simulink model "LowPassFilter_TEST"  (R2020a)
settings: Solver=VariableStepAuto  StartTime=0.0  StopTime=10.0  RelTol=1e-3
settings Model: Creator=109813  LastModifiedBy=109813

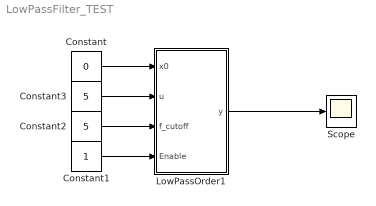
== system LowPassFilter_TEST ==
  Constant : Constant  Value=0
  Constant1 : Constant
  Constant2 : Constant  Value=5
  Constant3 : Constant  Value=5
  LowPassOrder1 : Subsystem
  Scope : Scope
  wires:
  Constant/1 -> LowPassOrder1/1(x0)
  Constant1/1 -> LowPassOrder1/4(Enable)
  Constant2/1 -> LowPassOrder1/3(f_cutoff)
  Constant3/1 -> LowPassOrder1/2(u)
  LowPassOrder1/1(y) -> Scope/1

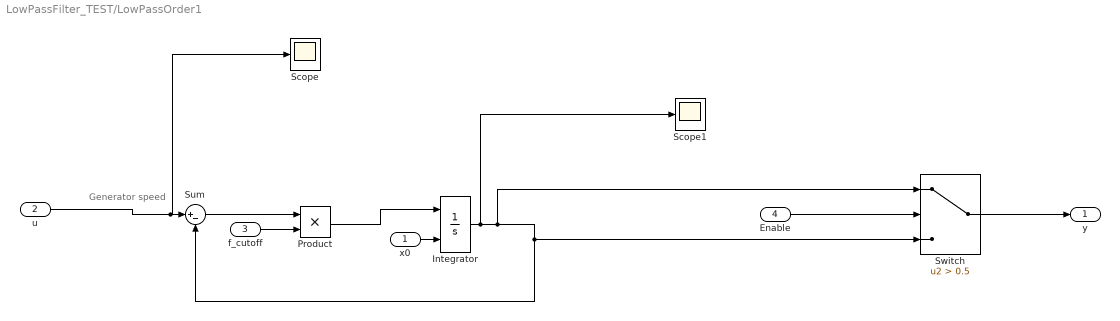
== system LowPassFilter_TEST/LowPassOrder1 ==
  note: Generator speed
  x0 : Inport
  u : Inport  Port=2
  f_cutoff : Inport  Port=3
  Enable : Inport  Port=4
  Integrator : Integrator  InitialConditionSource=external
  Product : Product
  Scope : Scope
  Scope1 : Scope
  Sum : Sum  Inputs=|+-
  Switch : Switch  Criteria=u2 > Threshold  Threshold=0.5
  y : Outport  VectorParamsAs1DForOutWhenUnconnected=off
  wires:
  Switch/1 -> y/1
  Enable/1 -> Switch/2
  f_cutoff/1 -> Product/2
  Product/1 -> Integrator/1
  u/1 -> Scope/1, Sum/1
  Integrator/1 -> Scope1/1, Switch/1, Sum/2, Switch/3
  Sum/1 -> Product/1
  x0/1 -> Integrator/2
